simulink model "kopter_se_zavazim_simulace_2024a"  (R2024a)
settings: Solver=FixedStepAuto  StartTime=0.0  StopTime=5  FixedStep=0.01  RelTol=1e-3
values from neighbouring files (symbols this model uses):
  b_moment = 5.4e-6    (= 5.4e-06)    [parametry_kopter_se_zavazim.m]
  d = 1    [parametry_kopter_se_zavazim.m]
  g = 9.81    [parametry_kopter_se_zavazim.m]
  Ip = m*d^2    (= 1)    [parametry_kopter_se_zavazim.m]
  Ixx = 0.0222    [parametry_kopter_se_zavazim.m]
  Iyy = 0.0222    [parametry_kopter_se_zavazim.m]
  Izz = 0.0429    [parametry_kopter_se_zavazim.m]
  k_thrust = 2.3e-3    (= 0.0023)    [parametry_kopter_se_zavazim.m]
  M = 2    [parametry_kopter_se_zavazim.m]
  m = 1    [parametry_kopter_se_zavazim.m]
  Us_p = [(M+m)*g; 0; 0; 0]    [parametry_kopter_se_zavazim.m]
  Xinit_matrix = [xyz_init; uhly_init; zavazi_init]    [parametry_kopter_se_zavazim.m]
  Xinit_ss = [Xinit_matrix; [0 0 0 0 0 0 0 0]']    [parametry_kopter_se_zavazim.m]
  Xs_p = [0;0;0; 0;0;0; 0;0; 0;0;0; 0;0;0; 0;0]    [parametry_kopter_se_zavazim.m]
undefined symbols (not defined in the file or in its folder): L
libraries: simulink_extras x6
(part 3 of 5)

== matlab function kopter_se_zavazim_simulace_2024a/Linearni State-Space (se zavazim) /MATLAB Function ==
  data: u output; m1 input; m2 input; m3 input; m4 input; k_thrust parameter; b_moment parameter; L parameter
function u = fcn(m1, m2, m3, m4, k_thrust, b_moment, L)

Thrust = k_thrust*(m1^2 + m2^2 + m3^2 + m4^2);
Tau_roll = L*k_thrust*(m1^2 + m4^2 - m2^2 - m3^2);
Tau_pitch = L*k_thrust*(m4^2 + m3^2 - m1^2 - m2^2);
Tau_yaw = b_moment*(m1^2 + m3^2 - m2^2 - m4^2);

u = [Thrust; Tau_roll; Tau_pitch; Tau_yaw];

== matlab function kopter_se_zavazim_simulace_2024a/Linearni State-Space (se zavazim) /Ac ==
  data: g parameter; M parameter; Ac output; m parameter; Ip parameter; d parameter
function Ac = fcn(g, M, m, Ip, d)
% Matice Ac linearizovana kvadrokoptera+zavazi

Ac = [
0, 0, 0,  0,                                                0, 0,                                        0, 0, 1, 0, 0, 0, 0, 0, 0, 0;
0, 0, 0,  0,                                                0, 0,                                        0, 0, 0, 1, 0, 0, 0, 0, 0, 0;
0, 0, 0,  0,                                                0, 0,                                        0, 0, 0, 0, 1, 0, 0, 0, 0, 0;
0, 0, 0,  0,                                                0, 0,                                        0, 0, 0, 0, 0, 1, 0, 0, 0, 0;
0, 0, 0,  0,                                                0, 0,                                        0, 0, 0, 0, 0, 0, 1, 0, 0, 0;
0, 0, 0,  0,                                                0, 0,                                        0, 0, 0, 0, 0, 0, 0, 1, 0, 0;
0, 0, 0,  0,                                                0, 0,                                        0, 0, 0, 0, 0, 0, 0, 0, 1, 0;
0, 0, 0,  0,                                                0, 0,                                        0, 0, 0, 0, 0, 0, 0, 0, 0, 1;
0, 0, 0,  0, (g*(M + m)*(m*d^2 + Ip))/(M*m*d^2 + Ip*m + Ip*M), 0,      (d^2*g*m^2)/(M*m*d^2 + Ip*m + Ip*M), 0, 0, 0, 0, 0, 0, 0, 0, 0;
0, 0, 0, -g,                                                0, 0,                                        0, 0, 0, 0, 0, 0, 0, 0, 0, 0;
0, 0, 0,  0,                                                0, 0,                                        0, 0, 0, 0, 0, 0, 0, 0, 0, 0;
0, 0, 0,  0,                                                0, 0,                                        0, 0, 0, 0, 0, 0, 0, 0, 0, 0;
0, 0, 0,  0,                                                0, 0,                                        0, 0, 0, 0, 0, 0, 0, 0, 0, 0;
0, 0, 0,  0,                                                0, 0,                                        0, 0, 0, 0, 0, 0, 0, 0, 0, 0;
0, 0, 0,  0,         -(d*g*m*(M + m))/(M*m*d^2 + Ip*m + Ip*M), 0, -(d*g*m*(M + m))/(M*m*d^2 + Ip*m + Ip*M), 0, 0, 0, 0, 0, 0, 0, 0, 0;
0, 0, 0,  0,                                                0, 0,                                        0, 0, 0, 0, 0, 0, 0, 0, 0, 0];

== matlab function kopter_se_zavazim_simulace_2024a/Maticovy popis (se zavazim)/C_G ==
  data: roll input; C_G output; pitch input; yaw input; alpha input; beta input; droll input; dpitch input; dyaw input; dalpha input; dbeta input; Ixx parameter; Iyy parameter; Izz parameter; d parameter; m parameter
function C_G = fcn(roll, pitch, yaw, alpha, beta, droll, dpitch, dyaw, dalpha, dbeta, Ixx, Iyy, Izz, d, m)
% Matice Coriolisovych sil a odporu vzduchu

phi_t = roll;
theta_t = pitch;
psi_t = yaw;

phi_dot_t = droll;
theta_dot_t = dpitch;
psi_dot_t = dyaw;

alpha_t = alpha;
beta_t = beta;

alpha_dot_t = dalpha;
beta_dot_t = dbeta;


C_G = [
0, 0, 0,                                                                                                                                                                                                                                                                    0,                                                                                                                                                                                                                                           0,                                                                                                                                   0,                                                         - alpha_dot_t*d*m*cos(beta_t)*sin(alpha_t) - 2*beta_dot_t*d*m*cos(alpha_t)*sin(beta_t),                                                                    -beta_dot_t*d*m*cos(beta_t)*sin(alpha_t);
0, 0, 0,                                                                                                                                                                                                                                                                    0,                                                                                                                                                                                                                                           0,                                                                                                                                   0,                                                           2*beta_dot_t*d*m*cos(alpha_t)*cos(beta_t) - alpha_dot_t*d*m*sin(alpha_t)*sin(beta_t),                                                                    -beta_dot_t*d*m*sin(alpha_t)*sin(beta_t);
0, 0, 0,                                                                                                                                                                                                                                                                    0,                                                                                                                                                                                                                                           0,                                                                                                                                   0,                                                                                                                   alpha_dot_t*d*m*cos(alpha_t),                                                                                                           0;
0, 0, 0,                                                                                                                                                                                                                                                                    0,          theta_dot_t*(Iyy*cos(phi_t)*sin(phi_t) - Izz*cos(phi_t)*sin(phi_t)) - psi_dot_t*(Ixx*cos(theta_t) + Iyy*cos(phi_t)^2*cos(theta_t) - Izz*cos(phi_t)^2*cos(theta_t) - Iyy*cos(theta_t)*sin(phi_t)^2 + Izz*cos(theta_t)*sin(phi_t)^2),                                    -psi_dot_t*(Iyy*cos(phi_t)*cos(theta_t)^2*sin(phi_t) - Izz*cos(phi_t)*cos(theta_t)^2*sin(phi_t)),                                                                                                                                              0,                                                                                                           0;
0, 0, 0,                               psi_dot_t*(Ixx*cos(theta_t) + Iyy*cos(phi_t)^2*cos(theta_t) - Izz*cos(phi_t)^2*cos(theta_t) - Iyy*cos(theta_t)*sin(phi_t)^2 + Izz*cos(theta_t)*sin(phi_t)^2) - theta_dot_t*(2*Iyy*cos(phi_t)*sin(phi_t) - 2*Izz*cos(phi_t)*sin(phi_t)),                                                                                                                                                                                                                                           0, psi_dot_t*(Izz*cos(phi_t)^2*cos(theta_t)*sin(theta_t) - Ixx*cos(theta_t)*sin(theta_t) + Iyy*cos(theta_t)*sin(phi_t)^2*sin(theta_t)),                                                                                                                                              0,                                                                                                           0;
0, 0, 0, psi_dot_t*(2*Iyy*cos(phi_t)*cos(theta_t)^2*sin(phi_t) - 2*Izz*cos(phi_t)*cos(theta_t)^2*sin(phi_t)) - theta_dot_t*(Ixx*cos(theta_t) - Iyy*cos(phi_t)^2*cos(theta_t) + Izz*cos(phi_t)^2*cos(theta_t) + Iyy*cos(theta_t)*sin(phi_t)^2 - Izz*cos(theta_t)*sin(phi_t)^2), - theta_dot_t*(Iyy*cos(phi_t)*sin(phi_t)*sin(theta_t) - Izz*cos(phi_t)*sin(phi_t)*sin(theta_t)) - psi_dot_t*(2*Izz*cos(phi_t)^2*cos(theta_t)*sin(theta_t) - 2*Ixx*cos(theta_t)*sin(theta_t) + 2*Iyy*cos(theta_t)*sin(phi_t)^2*sin(theta_t)),                                                                                                                                   0,                                                                                                                                              0,                                                                                                           0;
0, 0, 0,                                                                                                                                                                                                                                                                    0,                                                                                                                                                                                                                                           0,                                                                                                                                   0, -alpha_dot_t*(d^2*m*cos(alpha_t)*cos(beta_t)^2*sin(alpha_t) - d^2*m*cos(alpha_t)*sin(alpha_t) + d^2*m*cos(alpha_t)*sin(alpha_t)*sin(beta_t)^2), -beta_dot_t*(m*cos(alpha_t)*sin(alpha_t)*d^2*cos(beta_t)^2 + m*cos(alpha_t)*sin(alpha_t)*d^2*sin(beta_t)^2);
0, 0, 0,                                                                                                                                                                                                                                                                    0,                                                                                                                                                                                                                                           0,                                                                                                                                   0,                                 beta_dot_t*(2*d^2*m*cos(alpha_t)*cos(beta_t)^2*sin(alpha_t) + 2*d^2*m*cos(alpha_t)*sin(alpha_t)*sin(beta_t)^2),                                                                                                           0];

== matlab function kopter_se_zavazim_simulace_2024a/Maticovy popis (se zavazim)/inv(MM) ==
  data: roll input; invMM output; pitch input; yaw input; alpha input; beta input; M parameter; Ixx parameter; Iyy parameter; Izz parameter; d parameter; m parameter; Ip parameter
function invMM = fcn(roll, pitch, yaw, alpha, beta, M, Ixx, Iyy, Izz, d, m, Ip)
% Matice hmotnosti a setrvacnosti

phi_t = roll;
theta_t = pitch;
psi_t = yaw;

alpha_t = alpha;
beta_t = beta;

MM = [
                        M + m,                            0,                0,                 0,                                              0,                                                                                      0, d*m*cos(alpha_t)*cos(beta_t), -d*m*sin(alpha_t)*sin(beta_t);
                            0,                        M + m,                0,                 0,                                              0,                                                                                      0, d*m*cos(alpha_t)*sin(beta_t),  d*m*cos(beta_t)*sin(alpha_t);
                            0,                            0,            M + m,                 0,                                              0,                                                                                      0,             d*m*sin(alpha_t),                             0;
                            0,                            0,                0,               Ixx,                                              0,                                                                      -Ixx*sin(theta_t),                            0,                             0;
                            0,                            0,                0,                 0,      Iyy - Iyy*sin(phi_t)^2 + Izz*sin(phi_t)^2,                                         cos(phi_t)*cos(theta_t)*sin(phi_t)*(Iyy - Izz),                            0,                             0;
                            0,                            0,                0, -Ixx*sin(theta_t), cos(phi_t)*cos(theta_t)*sin(phi_t)*(Iyy - Izz), Izz*cos(phi_t)^2*cos(theta_t)^2 + Iyy*cos(theta_t)^2*sin(phi_t)^2 + Ixx*sin(theta_t)^2,                            0,                             0;
 d*m*cos(alpha_t)*cos(beta_t), d*m*cos(alpha_t)*sin(beta_t), d*m*sin(alpha_t),                 0,                                              0,                                                                                      0,                   m*d^2 + Ip,                             0;
-d*m*sin(alpha_t)*sin(beta_t), d*m*cos(beta_t)*sin(alpha_t),                0,                 0,                                              0,                                                                                      0,                            0,     m*d^2*sin(alpha_t)^2 + Ip];
 

invMM = inv(MM);

== matlab function kopter_se_zavazim_simulace_2024a/Maticovy popis (se zavazim)/Q ==
  data: alpha input; M parameter; Q output; g parameter; m parameter; d parameter
function Q = fcn(alpha, M, g, m, d)
alpha_t = alpha;
% Matice tihovych sil
Q = [0 0 (M+m)*g 0 0 0 d*g*m*sin(alpha_t) 0]';

== matlab function kopter_se_zavazim_simulace_2024a/Maticovy popis (se zavazim)/L ==
  data: roll input; L output; pitch input; yaw input
function L = fcn(roll, pitch, yaw)
% Matice vah vstupu

phi_t = roll;
theta_t = pitch;
psi_t = yaw;

L = [
sin(phi_t)*sin(psi_t) + cos(phi_t)*cos(psi_t)*sin(theta_t), 0, 0, 0;
cos(phi_t)*sin(psi_t)*sin(theta_t) - cos(psi_t)*sin(phi_t), 0, 0, 0;
                                   cos(phi_t)*cos(theta_t), 0, 0, 0;
                                                         0, 1, 0, 0;
                                                         0, 0, 1, 0;
                                                         0, 0, 0, 1;
                                                         0, 0, 0, 0;
                                                         0, 0, 0, 0];

== matlab function kopter_se_zavazim_simulace_2024a/Maticovy popis (se zavazim)/MATLAB Function ==
  data: u output; m1 input; m2 input; m3 input; m4 input; k_thrust parameter; b_moment parameter; L parameter
function u = fcn(m1, m2, m3, m4, k_thrust, b_moment, L)

Thrust = k_thrust*(m1^2 + m2^2 + m3^2 + m4^2);
Tau_roll = L*k_thrust*(m1^2 + m4^2 - m2^2 - m3^2);
Tau_pitch = L*k_thrust*(m4^2 + m3^2 - m1^2 - m2^2);
Tau_yaw = b_moment*(m1^2 + m3^2 - m2^2 - m4^2);

u = [Thrust; Tau_roll; Tau_pitch; Tau_yaw];
